simulink model "sim_init_example"  (Simulink 8.1)
settings: Solver=FixedStepDiscrete  StartTime=0.0  StopTime=5.0  FixedStep=1  RelTol=1e-3
settings Model: Creator=gcampa  LastModifiedBy=gcampa
settings OptimizationCC: ExpressionDepthLimit=128
settings DebuggingCC: FcnCallInpInsideContextMsg=EnableAllAsWarning

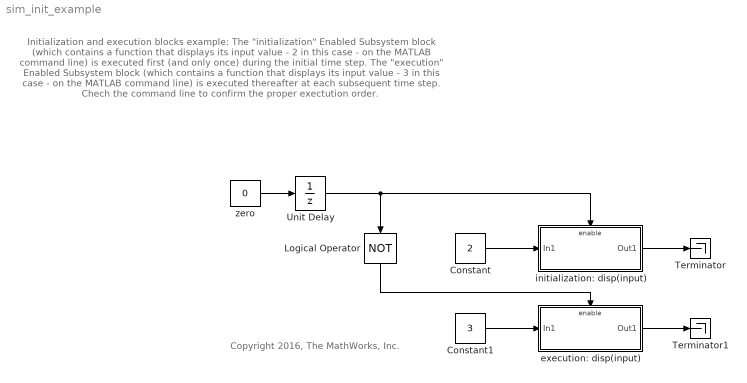
== system sim_init_example ==
  note: Initialization and execution blocks example:
      |
      | The "initialization" Enabled Subsystem block (which contains a function that displays its
      | input value - 2 in this case - on the MATLAB command line) is executed first (and only
      | once) during the initial time step.
      |
      | The "execution" Enabled Subsystem block (which contains a function that displays its
      | input value - 3 in this case - on the MATLAB command line) is executed thereafter at each
      | subsequent time step.
      |
      | Chech the command line to confirm the proper exectution order.
  note: Copyright 2016, The MathWorks, Inc.
  Constant : Constant  Value=2
  Constant1 : Constant  Value=3
  Logical Operator : Logic  Operator=NOT  AllPortsSameDT=off  OutDataTypeStr=boolean
  Terminator : Terminator
  Terminator1 : Terminator
  Unit Delay : UnitDelay  InitialCondition=1  SampleTime=-1
  execution: disp(input) : Subsystem  TreatAsAtomicUnit=on
  initialization: disp(input) : Subsystem  TreatAsAtomicUnit=on
  zero : Constant  Value=0
  wires:
  zero/1 -> Unit Delay/1
  Unit Delay/1 -> initialization: disp(input)/Enable, Logical Operator/1
  Constant/1 -> initialization: disp(input)/1(In1)
  Logical Operator/1 -> execution: disp(input)/Enable
  Constant1/1 -> execution: disp(input)/1(In1)
  initialization: disp(input)/1(Out1) -> Terminator/1
  execution: disp(input)/1(Out1) -> Terminator1/1

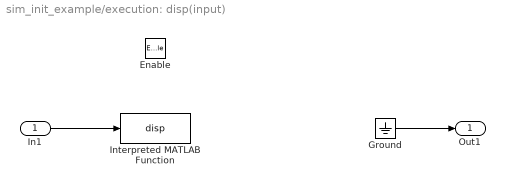
== system sim_init_example/execution: disp(input) ==
  In1 : Inport
  Enable : EnablePort
  Ground : Ground
  Interpreted MATLAB Function : MATLABFcn  MATLABFcn=disp  OutputDimensions=0
  Out1 : Outport
  wires:
  Ground/1 -> Out1/1
  In1/1 -> Interpreted MATLAB Function/1

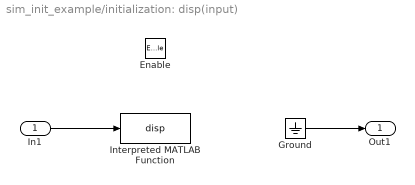
== system sim_init_example/initialization: disp(input) ==
  In1 : Inport
  Enable : EnablePort
  Ground : Ground
  Interpreted MATLAB Function : MATLABFcn  MATLABFcn=disp  OutputDimensions=0
  Out1 : Outport
  wires:
  In1/1 -> Interpreted MATLAB Function/1
  Ground/1 -> Out1/1
